simulink model "photoin"  (R2014b)
settings: Solver=ode45  StartTime=0.0  StopTime=10.0  RelTol=1e-3
undefined symbols (not defined in the file or in its folder): Rec, SDTV
libraries: visionconversions x1, visionsources x1
settings Model: Creator=Jackie  LastModifiedBy=Jackie

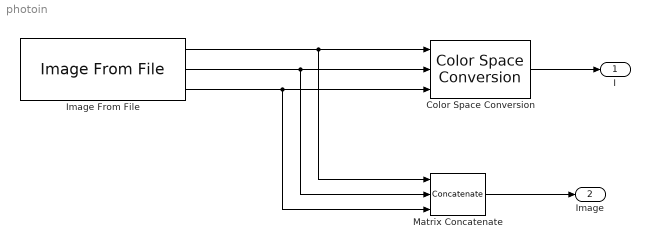
== system photoin ==
  Color Space Conversion : visionconversions/Color Space  Conversion  conversion=Obsolete  conversionActive=R'G'B' to intensity  wp_str=D65  rec=Rec. 601 (SDTV)  sys=1125/60/2:1  imagePorts=Separate color signals
  Image From File : visionsources/Image From File  Tag=vipblks_nd  FileName=test1.jpg  imagePorts=Separate color signals  Ts=inf  ImageDataType=single  Signed=on  WordLength=16  sdImageDataType=uint(8)  FractionLengthMode=User-defined  FractionLength=15  OutPortLabels=R|G|B
  Matrix Concatenate : Concatenate  NumInputs=3  Mode=Multidimensional array  ConcatenateDimension=2
  I : Outport
  Image : Outport  Port=2
  wires:
  Matrix Concatenate/1 -> Image/1
  Color Space Conversion/1 -> I/1
  Image From File/1 -> Matrix Concatenate/1, Color Space Conversion/1
  Image From File/2 -> Matrix Concatenate/2, Color Space Conversion/2
  Image From File/3 -> Matrix Concatenate/3, Color Space Conversion/3
